simulink model "bm99exp"  (Simulink 7.3)
settings: Solver=ode45  StartTime=0.0  StopTime=Tstop  RelTol=1e-3
values from neighbouring files (symbols this model uses):
  E = expcon(C,range,options)    [bm99benchmark.m]    (also in bm99norm2.m; bm99sim.m; heatcool.m; hybexp3.m)
libraries: hyblib x2
settings Model: Creator=Alberto Bemporad  LastModifiedBy=Alberto Bemporad
settings DataIOCC: SignalLoggingName=sigsOut
settings DebuggingCC: SaveWithParameterizedLinksMsg=none  SignalResolutionControl=TryResolveAllWithWarning  SolverPrmCheckMsg=none  MultiTaskDSMMsg=warning  MultiTaskCondExecSysMsg=none  StrictBusMsg=None
settings HardwareCC: TargetUnknown=on
settings RTWCC: IncludeERTFirstTime=on

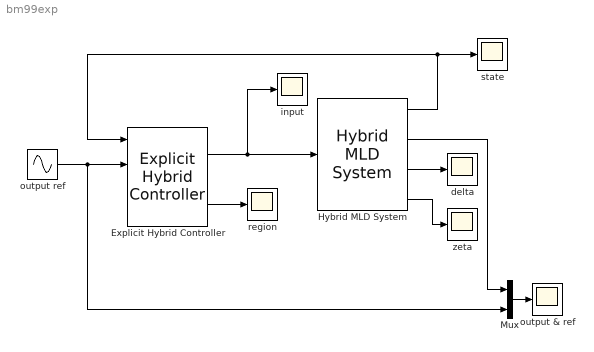
== system bm99exp ==
  Explicit Hybrid Controller : hyblib/Explicit Hybrid Controller  SystemSampleTime=-1  C=E  compile=on
  Hybrid MLD System : hyblib/Hybrid MLD System  SystemSampleTime=-1  S=S  x0init=x0
  Mux : Mux  Inputs=2
  delta : Scope
  input : Scope
      settings: TimeRange=100  YMin=-1  YMax=0.4  SaveName=ScopeData2
  output & ref : Scope
      settings: TimeRange=100  YMin=-1  YMax=1  SaveName=ScopeData4
  output ref : Sin  Amplitude=1  Bias=0  Frequency=1/8  Phase=0  Samples=10  SampleTime=0  Offset=0
  region : Scope
      settings: TimeRange=100  YMin=1  SaveName=ScopeData5
  state : Scope
      settings: SaveName=ScopeData3
  zeta : Scope
  wires:
  Explicit Hybrid Controller/1 -> input/1, Hybrid MLD System/1
  output ref/1 -> Mux/2, Explicit Hybrid Controller/2
  Mux/1 -> output & ref/1
  Hybrid MLD System/1 -> state/1, Explicit Hybrid Controller/1
  Explicit Hybrid Controller/2 -> region/1
  Hybrid MLD System/2 -> Mux/1
  Hybrid MLD System/4 -> zeta/1
  Hybrid MLD System/3 -> delta/1
